simulink library "passive_control"  (Simulink 7.1)
values from neighbouring files (symbols this model uses):
  sysdsp = feedback(sysdp,Kc)    [calc_sysdsp.m]
  Ts = 1    [calc_sysdsp.m]
undefined symbols (not defined in the file or in its folder): A, B, b, C, D, gravload, Kv, Kx, M, ms, nc, np, q0, tau_passify
libraries: instrumentlib x8, passive_control x4, simulink x4, roblocks x2, dspsigops x2
(part 1 of 2)
settings Model: Creator=Administrator  LastModifiedBy=Tilt_Press

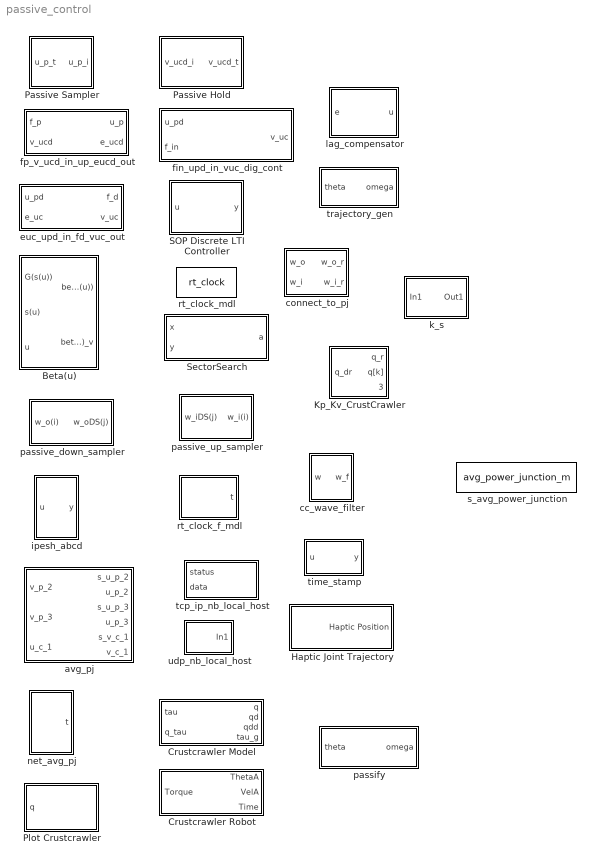
== system passive_control ==
  Beta(u) : Subsystem  mask{n=1}
      mask prompts: n "Enter Length of u"
  Crustcrawler Model : Subsystem  mask{q0=[0,-pi/2,pi/2,0]}
      mask prompts: q0 "Initial State [q0]"
      mask init:
      | srobot = crust_crawler_robot();
  Crustcrawler Robot : Subsystem  mask{Ts=0}
      mask prompts: Ts "Enter Ts"
  Haptic Joint Trajectory : Subsystem  SystemSampleTime=.04
  Kp_Kv_CrustCrawler : Subsystem  mask{q0=q0, Ts=Ts, Kv=Kv, Kx=Kx, Kg_on=off, b=b}
      mask prompts: q0 "Initial State (radians) [q0]"; Ts "Sample Rate (s) [Ts]"; Kv "Velocity Loop Gain [Kv]"; Kx "Position Loop Gain [Kx]"; Kg_on "Gravity Comp On [Kg] {0,1}"; b "wave impedance [b]"
      mask init:
      | if Kg_on
      |     Kg=1;
      | else
      |     Kg=0;
      | end
  Passive Hold : Subsystem  mask{Ts=.05}
      mask prompts: Ts "Hold Time (seconds):"
  Passive Sampler : Subsystem  mask{Ts=.05}
      mask prompts: Ts "Sample Time (seconds):"
  Plot Crustcrawler : Subsystem
      mask init:
      | srobot = crust_crawler_robot();
  SOP Discrete LTI Controller : Subsystem  mask{Kp=1, Kd=1, Kc=1.0e-6, x0=0, Ts=.05}
      mask prompts: Kp "Enter Kp (Kp > 0), (Kp in R^(mxm)):"; Kd "Enter Kd (Kd > 0), (Kd in R^(mxm)):"; Kc "Enter SOP feedback gain (Kc)"; x0 "Initial Conditions:"; Ts "Enter Sample Time (seconds):"
      mask help:
      | This will implement a (strictly) output passive digital controller
      | (if Kc > 0) based on its continuous passive PD controller counterpart.
      | The user just needs to insure that Kp > 0 and Kd > 0 (are positive
      | definite matrices).  For simplicity Kc can be a scalar.
      mask init:
      | [x0,sysdsp]=calc_sysdsp(Kp,Kd,Kc,x0,Ts);
  SectorSearch : Subsystem
  avg_pj : Subsystem  Orientation=left  mask{np=2, nc=1, ms=3, Ts=.05}
      mask prompts: np "Enter Number of Plants [np]"; nc "Enter Number of Controllers [nc]"; ms "Enter Vector Length [ms]"; Ts "Enter Sample Time (s) [Ts]"
  cc_wave_filter : Subsystem  mask{wn=1, Ts=.04}
      mask prompts: wn "Enter wn [wn] (rad/sec)"; Ts "Enter Sample rate [Ts] (sec)"
  connect_to_pj : Subsystem  mask{connect=on}
  euc_upd_in_fd_vuc_out : Subsystem  mask{b=1}
      mask prompts: b "Enter b:"
  fin_upd_in_vuc_dig_cont : Subsystem  mask{Kp=1, Kd=1, Kc=1.0e-6, b=1, x0=0, Ts=.05}
      mask prompts: Kp "Enter Kp (Kp > 0), (Kp in R^(mxm)):"; Kd "Enter Kd (Kd > 0), (Kd in R^(mxm)):"; Kc "Enter SOP feedback gain (Kc):"; b "Enter b:"; x0 "Initial Conditions:"; Ts "Enter Sample Time (seconds):"
      mask init:
      | [x0,sysdsp]=calc_sysdsp(Kp,Kd,Kc,x0,Ts);
      | sysdsp_ib=feedback(sysdsp,(1/b)*eye(size(sysdsp.d)));
  fp_v_ucd_in_up_eucd_out : Subsystem  mask{b=1}
      mask prompts: b "Enter b:"
  ipesh_abcd : Subsystem  mask{num=[1 0], den=[.02/pi 1], Ts=.02}
      mask prompts: num "Enter num of H(s) [num]"; den "Enter den of H(s) [den]"; Ts "Enter sample time (s) [Ts]"
      mask init:
      | Hs=tf(num,den);
      | Hz=ipesh_transform(Hs,Ts);
      | [A,B,C,D]=tf2ss(Hz.num{1},Hz.den{1});
      | [m,n]=size(A);
      | x0=zeros(1,n);
  k_s : Subsystem  mask{M=2, n_p=2}
      mask prompts: M "Enter Upsample / Downsample [M]"; n_p "Enter number of plants"
      mask init:
      | m=1;
      | n=n_p+m;
      | k_s=sqrt(M)*sqrt((n-m))/sqrt(m);
  lag_compensator : Subsystem  mask{K=.5, omega=pi/2, Ts=2*.04}
      mask prompts: omega "omega (rad/sec) [omega]"; Ts "sample rate (s) [Ts]"
  net_avg_pj : Subsystem  mask{udp_start_port=9000, Ts=.05, max_pc=100, ID=1}
      mask prompts: udp_start_port "Enter UDP Start Port [udp_start_port]"; Ts "Enter PJ Sample Time [Ts]"; max_pc "Enter max_pc [max_pc]"; ID "Enter time ID [ID]"
      mask CallbackString:
      | udp_start_port=eval(get_param(gcb,'udp_start_port'));
      | max_pc=eval(get_param(gcb,'max_pc'));
      | Ts=eval(get_param(gcb,'Ts'));
      | for i = 2:3
      |     obj=[gcb,'/Plant_',num2str(i),'_u'];
      |     set_param(obj,'port',num2str(udp_start_port+max_pc+i-1));
      |     set_param(obj,'Ts',num2str(Ts));
      |     obj=[gcb,'/Plant_',num2str(i),'_v'];
      |     set_param(obj,'port',num2str(udp_start_port+2*max_pc+i-1));
      | end
      | set_param([gcb,'/Controller_1_v'],'port',num2str(udp_start_port+max_pc));
      | set_param([gcb,'/Controller_1_v'],'Ts',num2str(Ts));
      | set_param([gcb,'/Controller_1_u'],'port',num2str(udp_start_port+2*max_pc));
      | |||
  passify : Subsystem  mask{tau=tau_passify, Ts=Ts}
      mask prompts: tau "tau (seconds) [tau]"; Ts "Sample rate (seconds) Ts"
  passive_down_sampler : Subsystem  mask{M=M}
      mask prompts: M "Enter Downsample Integer M:"
  passive_up_sampler : Subsystem  mask{M=2, N=2}
      mask prompts: M "Enter Upsampler Integer M:"; N "Dimension of Input Vector N:"
  rt_clock_f_mdl : Subsystem  mask{Ts=.05, ID=1}
      mask prompts: Ts "Enter Step Size (seconds)"; ID "Enter Timer ID {1,2,...}"
  rt_clock_mdl : S-Function  FunctionName=rt_clock  Parameters=1,.05  EnableBusSupport=off
  s_avg_power_junction : S-Function  FunctionName=avg_power_junction_m  Parameters=ms,np,nc,Ts  EnableBusSupport=off
  tcp_ip_nb_local_host : Subsystem  Orientation=left  mask{port=10000, ms=3, Ts=.05}
      mask prompts: port "Port: [port]"; ms "Vector length: [ms]"; Ts "Block sample time: [Ts]"
      mask CallbackString:
      | port=eval(get_param(gcb,'port'));
      | set_param([gcb,'/tcp_ip_r'],'Port',num2str(port));
      | |ms=eval(get_param(gcb,'ms'));
      | set_param([gcb,'/tcp_ip_r'],'DataSize',['[',num2str(ms),']']);|Ts=eval(get_param(gcb,'Ts'));
      | set_param([gcb,'/tcp_ip_r'],'SampleTime',num2str(Ts));
  time_stamp : Subsystem
      mask Description:
      | Adds return from clock to vector, to plot results which
      | were stored to file plant.mat for example do the following:
      | fh=load('plant');
      | t=fh.ans(1,:);
      | c_v=fh.ans(2:7,:);
      | theta=fh.ans(8:11,:);
      | t_ts=0*t;
      | i=1;
      | c_0=c_v(:,1);
      | for c = c_v
      |     t_ts(i) = etime(c',c_0');
      |     i = i + 1;
      | end
      | plot(t_ts,t-t_ts,t_ts,theta);grid;
  trajectory_gen : Subsystem  mask{zeta=.9, wn=2*pi/10, Ts=2*.04}
      mask prompts: zeta "zeta [zeta]"; wn "wn [wn] (rad/sec)"; Ts "sample rate (s) [Ts]"
  udp_nb_local_host : Subsystem  Orientation=left  mask{port=9001}
      mask prompts: port "Port: [port]"
      mask CallbackString:
      | port=eval(get_param(gcb,'port'));
      | set_param([gcb,'/udp_s'],'Port',num2str(port));

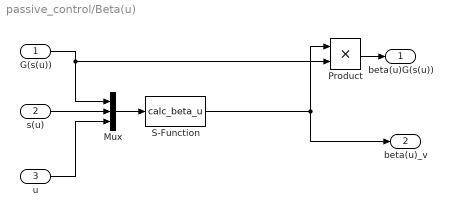
== system passive_control/Beta(u) ==
  G(s(u)) : Inport  OutDataType=sfix(16)  OutScaling=2^0
  s(u) : Inport  Port=2  OutDataType=sfix(16)  OutScaling=2^0
  u : Inport  Port=3  OutDataType=sfix(16)  OutScaling=2^0
  Mux : Mux  Inputs=3
  Product : Product  OutDataType=sfix(16)  OutScaling=2^0  RndMeth=Zero
  S-Function : S-Function  FunctionName=calc_beta_u  Parameters=n  EnableBusSupport=off
  beta(u)G(s(u)) : Outport  OutDataType=sfix(16)  OutScaling=2^0
  beta(u)_v : Outport  Port=2  OutDataType=sfix(16)  OutScaling=2^0
  wires:
  Product/1 -> beta(u)G(s(u))/1
  Mux/1 -> S-Function/1
  u/1 -> Mux/3
  s(u)/1 -> Mux/2
  G(s(u))/1 -> Product/2, Mux/1
  S-Function/1 -> Product/1, beta(u)_v/1

== system passive_control/Crustcrawler Model ==
  tau : Inport  OutDataType=sfix(16)  OutScaling=2^0
  q_tau : Inport  Port=2  OutDataType=sfix(16)  OutScaling=2^0
  Robot : roblocks/Robot  SystemSampleTime=-1  robot=srobot  q0=q0
      link override Integrator1: InitialCondition=q0
  gravity_compensation : MATLABFcn  MATLABFcn=gravload(srobot, u(1:4)')  OutputDimensions=4
  q : Outport  OutDataType=sfix(16)  OutScaling=2^0
  qd : Outport  Port=2  OutDataType=sfix(16)  OutScaling=2^0
  qdd : Outport  Port=3  OutDataType=sfix(16)  OutScaling=2^0
  tau_g : Outport  Port=4  OutDataType=sfix(16)  OutScaling=2^0
  wires:
  q_tau/1 -> gravity_compensation/1
  gravity_compensation/1 -> tau_g/1
  tau/1 -> Robot/1
  Robot/1 -> q/1
  Robot/2 -> qd/1
  Robot/3 -> qdd/1

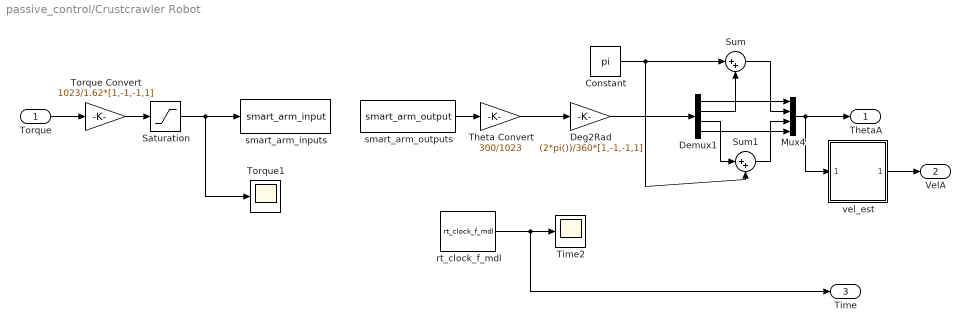
== system passive_control/Crustcrawler Robot ==
  Torque : Inport
  Constant : Constant  Value=pi  OutDataType=sfix(16)  OutScaling=2^0  SampleTime=Ts
  Deg2Rad : Gain  Gain=(2*pi())/360*[1,-1,-1,1]  ParameterDataType=sfix(16)  ParameterScaling=2^0  OutDataType=sfix(16)  OutScaling=2^0
  Demux1 : Demux
  Mux4 : Mux
  Saturation : Saturate  UpperLimit=1023  LowerLimit=-1023  OutDataType=sfix(16)  OutScaling=2^0
  Sum : Sum  Inputs=|++  OutDataType=sfix(16)  OutScaling=2^0
  Sum1 : Sum  Inputs=|++  OutDataType=sfix(16)  OutScaling=2^0
  Theta Convert : Gain  Gain=300/1023  ParameterDataType=sfix(16)  ParameterScaling=2^0  OutDataType=sfix(16)  OutScaling=2^0
  Time2 : Scope
      settings: TimeRange=100  YMin=-0.0275  YMax=0.02
  Torque Convert : Gain  Gain=1023/1.62*[1,-1,-1,1]  ParameterDataType=sfix(16)  ParameterScaling=2^0  OutDataType=sfix(16)  OutScaling=2^0
  Torque1 : Scope
      settings: TimeRange=100  YMin=-175  YMax=375
  rt_clock_f_mdl : passive_control/rt_clock_f_mdl  SystemSampleTime=-1  Ts=Ts  ID=1
  smart_arm_inputs : S-Function  Priority=1  FunctionName=smart_arm_input  Parameters=1, Ts  EnableBusSupport=off
  smart_arm_outputs : S-Function  Priority=2  FunctionName=smart_arm_output  Parameters=1, Ts  EnableBusSupport=off
  vel_est : Subsystem
  ThetaA : Outport
  VelA : Outport  Port=2
  Time : Outport  Port=3
  wires:
  vel_est/1(omega) -> VelA/1
  rt_clock_f_mdl/1 -> Time/1, Time2/1
  Torque/1 -> Torque Convert/1
  Theta Convert/1 -> Deg2Rad/1
  Torque Convert/1 -> Saturation/1
  Mux4/1 -> vel_est/1(theta), ThetaA/1
  Demux1/1 -> Mux4/1
  Demux1/4 -> Mux4/4
  Deg2Rad/1 -> Demux1/1
  Sum/1 -> Mux4/2
  Constant/1 -> Sum/1, Sum1/2
  Demux1/2 -> Sum/2
  Demux1/3 -> Sum1/1
  Sum1/1 -> Mux4/3
  smart_arm_outputs/1 -> Theta Convert/1
  Saturation/1 -> Torque1/1, smart_arm_inputs/1

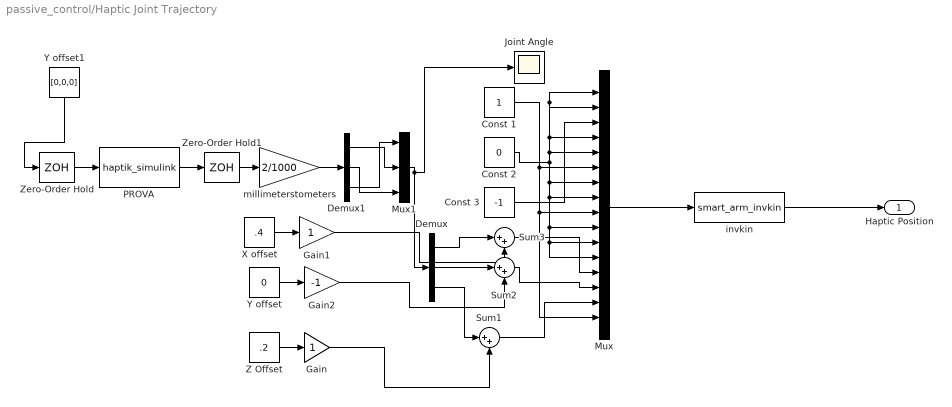
== system passive_control/Haptic Joint Trajectory ==
  Const 1 : Constant  OutDataType=sfix(16)  OutScaling=2^0
  Const 2 : Constant  Value=0  OutDataType=sfix(16)  OutScaling=2^0
  Const 3 : Constant  Value=-1  OutDataType=sfix(16)  OutScaling=2^0
  Demux : Demux  Outputs=3
  Demux1 : Demux  Outputs=3
  Gain : Gain  ParameterDataType=sfix(16)  ParameterScaling=2^0  OutDataType=sfix(16)  OutScaling=2^0
  Gain1 : Gain  ParameterDataType=sfix(16)  ParameterScaling=2^0  OutDataType=sfix(16)  OutScaling=2^0
  Gain2 : Gain  Gain=-1  ParameterDataType=sfix(16)  ParameterScaling=2^0  OutDataType=sfix(16)  OutScaling=2^0
  Joint Angle : Scope
      settings: TimeRange=100  YMin=-0.06  YMax=0.015
  Mux : Mux  Inputs=16
  Mux1 : Mux  Inputs=3
  PROVA : S-Function  FunctionName=haptik_simulink  EnableBusSupport=off
  Sum1 : Sum  Inputs=|++  OutDataType=sfix(16)  OutScaling=2^0
  Sum2 : Sum  Inputs=|++  OutDataType=sfix(16)  OutScaling=2^0
  Sum3 : Sum  Inputs=|++  OutDataType=sfix(16)  OutScaling=2^0
  X offset : Constant  Value=.4  OutDataType=sfix(16)  OutScaling=2^0
  Y offset : Constant  Value=0  OutDataType=sfix(16)  OutScaling=2^0
  Y offset1 : Constant  Orientation=down  Value=[0,0,0]  OutDataType=sfix(16)  OutScaling=2^0
  Z Offset : Constant  Value=.2  OutDataType=sfix(16)  OutScaling=2^0
  Zero-Order Hold : ZeroOrderHold  SampleTime=.04
  Zero-Order Hold1 : ZeroOrderHold  SampleTime=.04
  invkin : S-Function  FunctionName=smart_arm_invkin  Parameters=1  EnableBusSupport=off
  millimeterstometers : Gain  Gain=2/1000  ParameterDataType=sfix(16)  ParameterScaling=2^0  OutDataType=sfix(16)  OutScaling=2^0
  Haptic Position : Outport  OutDataType=sfix(16)  OutScaling=2^0
  wires:
  Gain1/1 -> Sum3/2
  Sum3/1 -> Mux/13
  Demux/1 -> Sum3/1
  X offset/1 -> Gain1/1
  Gain2/1 -> Sum2/2
  Sum2/1 -> Mux/14
  Demux/2 -> Sum2/1
  Mux1/1 -> Joint Angle/1, Demux/1
  millimeterstometers/1 -> Demux1/1
  Mux/1 -> invkin/1
  Const 2/1 -> Mux/4, Mux/1, Mux/2, Mux/5, Mux/8, Mux/10, Mux/12, Mux/11, Mux/7
  Const 1/1 -> Mux/6, Mux/16, Mux/9
  Sum1/1 -> Mux/15
  Gain/1 -> Sum1/2
  Demux/3 -> Sum1/1
  Z Offset/1 -> Gain/1
  Y offset/1 -> Gain2/1
  PROVA/1 -> Zero-Order Hold1/1
  Const 3/1 -> Mux/3
  Demux1/2 -> Mux1/3
  Demux1/1 -> Mux1/2
  Demux1/3 -> Mux1/1
  Zero-Order Hold/1 -> PROVA/1
  Zero-Order Hold1/1 -> millimeterstometers/1
  Y offset1/1 -> Zero-Order Hold/1
  invkin/1 -> Haptic Position/1

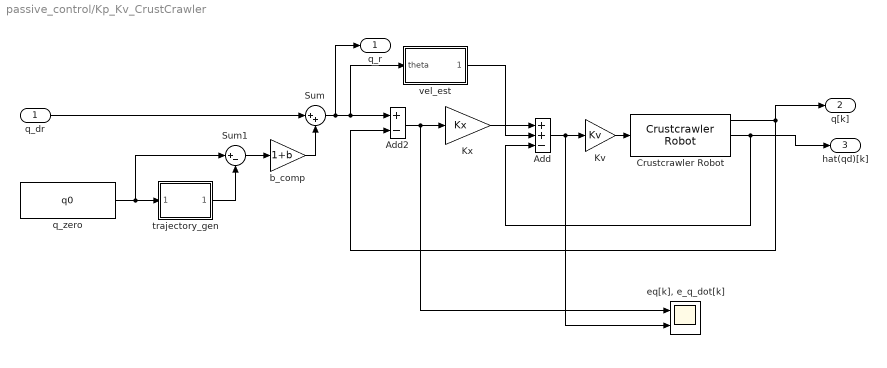
== system passive_control/Kp_Kv_CrustCrawler ==
  q_dr : Inport
  Add : Sum  Inputs=++-  OutDataType=sfix(16)  OutScaling=2^-10
  Add2 : Sum  Inputs=+-  OutDataType=sfix(16)  OutScaling=2^-10
  Crustcrawler Robot : passive_control/Crustcrawler Robot  SystemSampleTime=-1  Ts=Ts
  Kv : Gain  Gain=Kv  ParameterDataType=sfix(16)  ParameterScaling=2^0  OutDataType=sfix(16)  OutScaling=2^0
  Kx : Gain  Gain=Kx  ParameterDataType=sfix(16)  ParameterScaling=2^0  OutDataType=sfix(16)  OutScaling=2^0
  Sum : Sum  Inputs=|++  OutDataType=sfix(16)  OutScaling=2^0
  Sum1 : Sum  Inputs=|+-  OutDataType=sfix(16)  OutScaling=2^0
  b_comp : Gain  Gain=1+b  ParameterDataType=sfix(16)  ParameterScaling=2^0  OutDataType=sfix(16)  OutScaling=2^0
  "eq[k], e_q_dot[k]" : Scope  NumInputPorts=2
      settings: TimeRange=5  YMin=-0.01~-0.2  YMax=0.035~1  SaveName=ScopeData5
  q_zero : Constant  Value=q0  OutDataType=sfix(16)  OutScaling=2^0  SampleTime=0.04
  trajectory_gen : Subsystem  mask{zeta=.9, wn=2*pi/10, Ts=Ts}
      mask prompts: zeta "zeta [zeta]"; wn "wn [wn] (rad/sec)"; Ts "sample rate (s) [Ts]"
  vel_est : Subsystem  Priority=-1  mask{Ts=Ts, q0=q0*(1+b)}
      mask prompts: Ts "Enter Sample Rate [Ts] (seconds)"; q0 "Enter Initial State [q0] (radians)"
  q_r : Outport
  q[k] : Outport  Port=2
  hat(qd)[k] : Outport  Port=3
  wires:
  vel_est/1(omega) -> Add/2
  q_dr/1 -> Sum/1
  Crustcrawler Robot/2 -> hat(qd)[k]/1, Add/3
  Crustcrawler Robot/1 -> q[k]/1, Add2/2
  Sum/1 -> q_r/1, vel_est/1(theta), Add2/1
  Add/1 -> "eq[k], e_q_dot[k]"/2, Kv/1
  Kv/1 -> Crustcrawler Robot/1
  Kx/1 -> Add/1
  Add2/1 -> "eq[k], e_q_dot[k]"/1, Kx/1
  trajectory_gen/1(omega) -> Sum1/2
  q_zero/1 -> Sum1/1, trajectory_gen/1(theta)
  Sum1/1 -> b_comp/1
  b_comp/1 -> Sum/2

== system passive_control/Passive Hold ==
  v_ucd_i : Inport  OutDataType=sfix(16)  OutScaling=2^0
  Gain : Gain  Gain=1/sqrt(Ts)  ParameterDataType=sfix(16)  ParameterScaling=2^0  OutDataType=sfix(16)  OutScaling=2^0
  Zero-Order Hold : ZeroOrderHold  SampleTime=Ts
  v_ucd_t : Outport  OutDataType=sfix(16)  OutScaling=2^0
  wires:
  Zero-Order Hold/1 -> Gain/1
  Gain/1 -> v_ucd_t/1
  v_ucd_i/1 -> Zero-Order Hold/1

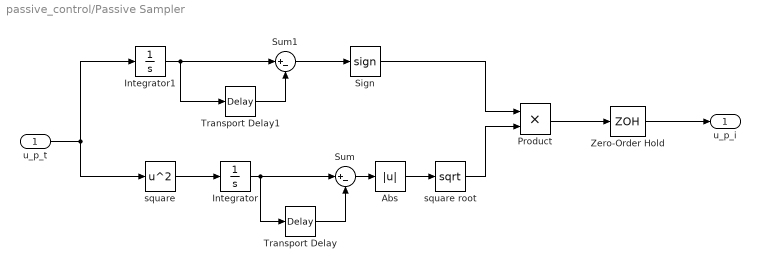
== system passive_control/Passive Sampler ==
  u_p_t : Inport  OutDataType=sfix(16)  OutScaling=2^0
  Abs : Abs  OutDataType=sfix(16)  OutScaling=2^0
  Integrator : Integrator
  Integrator1 : Integrator
  Product : Product  OutDataType=sfix(16)  OutScaling=2^0  RndMeth=Zero
  Sign : Signum
  Sum : Sum  Inputs=|+-  OutDataType=sfix(16)  OutScaling=2^0
  Sum1 : Sum  Inputs=|+-  OutDataType=sfix(16)  OutScaling=2^0
  Transport Delay : TransportDelay  DelayTime=Ts
  Transport Delay1 : TransportDelay  DelayTime=Ts
  Zero-Order Hold : ZeroOrderHold  SampleTime=Ts
  square : Math  Operator=square  OutDataType=sfix(16)  OutScaling=2^0  SaturateOnIntegerOverflow=on
  square root : Math  Operator=sqrt  OutDataType=sfix(16)  OutScaling=2^0  SaturateOnIntegerOverflow=on
  u_p_i : Outport  OutDataType=sfix(16)  OutScaling=2^0
  wires:
  Transport Delay/1 -> Sum/2
  Transport Delay1/1 -> Sum1/2
  Zero-Order Hold/1 -> u_p_i/1
  Sum1/1 -> Sign/1
  Integrator1/1 -> Sum1/1, Transport Delay1/1
  Sum/1 -> Abs/1
  Integrator/1 -> Transport Delay/1, Sum/1
  Sign/1 -> Product/1
  square root/1 -> Product/2
  square/1 -> Integrator/1
  u_p_t/1 -> square/1, Integrator1/1
  Abs/1 -> square root/1
  Product/1 -> Zero-Order Hold/1

== system passive_control/Plot Crustcrawler ==
  q : Inport  OutDataType=sfix(16)  OutScaling=2^0
  plot : roblocks/plot  SystemSampleTime=-1  robot=srobot
  wires:
  q/1 -> plot/1

== system passive_control/SOP Discrete LTI Controller ==
  u : Inport  OutDataType=sfix(16)  OutScaling=2^0
  Discrete State-Space : DiscreteStateSpace  A=sysdsp.a  B=sysdsp.b  C=sysdsp.c  D=sysdsp.d  X0=x0  SampleTime=-1
  y : Outport  OutDataType=sfix(16)  OutScaling=2^0
  wires:
  u/1 -> Discrete State-Space/1
  Discrete State-Space/1 -> y/1

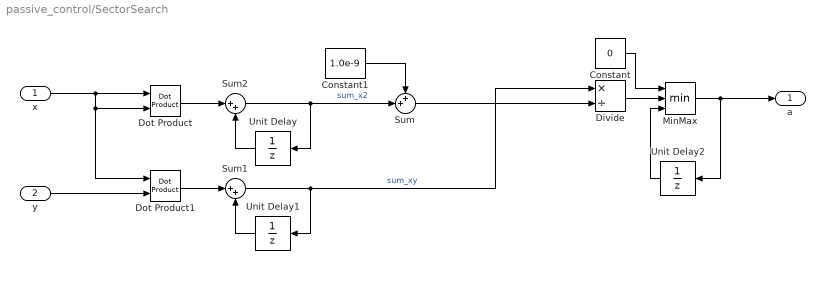
== system passive_control/SectorSearch ==
  x : Inport  OutDataType=sfix(16)  OutScaling=2^0
  y : Inport  Port=2  OutDataType=sfix(16)  OutScaling=2^0
  Constant : Constant  Value=0  OutDataType=sfix(16)  OutScaling=2^0
  Constant1 : Constant  Value=1.0e-9  OutDataType=sfix(16)  OutScaling=2^0
  Divide : Product  Inputs=*/  OutDataType=sfix(16)  OutScaling=2^-10
  Dot Product : simulink/Math Operations/Dot Product  InputSameDT=on  OutDataType=sfix(16)  OutScaling=2^-10  DoSatur=off
  Dot Product1 : simulink/Math Operations/Dot Product  InputSameDT=on  OutDataType=sfix(16)  OutScaling=2^-10  DoSatur=off
  MinMax : MinMax  Inputs=3  OutDataType=sfix(16)  OutScaling=2^0
  Sum : Sum  Inputs=++|  OutDataType=sfix(16)  OutScaling=2^0
  Sum1 : Sum  Inputs=|++  OutDataType=sfix(16)  OutScaling=2^0
  Sum2 : Sum  Inputs=|++  OutDataType=sfix(16)  OutScaling=2^0
  Unit Delay : UnitDelay  Orientation=left  SampleTime=-1
  Unit Delay1 : UnitDelay  Orientation=left  SampleTime=-1
  Unit Delay2 : UnitDelay  Orientation=left  SampleTime=-1
  a : Outport  OutDataType=sfix(16)  OutScaling=2^0
  wires:
  Sum2/1 -> Unit Delay/1, Sum/2  "sum_x2"
  Unit Delay/1 -> Sum2/2
  Dot Product/1 -> Sum2/1
  Sum1/1 -> Unit Delay1/1, Divide/1  "sum_xy"
  Unit Delay1/1 -> Sum1/2
  Dot Product1/1 -> Sum1/1
  x/1 -> Dot Product/1, Dot Product/2, Dot Product1/1
  y/1 -> Dot Product1/2
  MinMax/1 -> Unit Delay2/1, a/1
  Constant/1 -> MinMax/1
  Divide/1 -> MinMax/2
  Unit Delay2/1 -> MinMax/3
  Sum/1 -> Divide/2
  Constant1/1 -> Sum/1

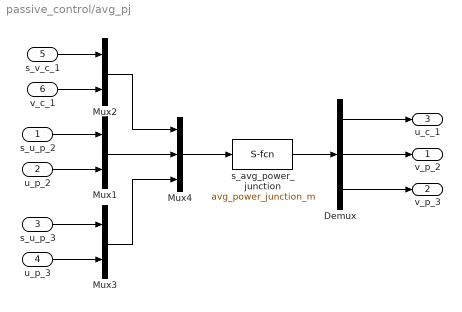
== system passive_control/avg_pj ==
  s_u_p_2 : Inport
  u_p_2 : Inport  Port=2
  s_u_p_3 : Inport  Port=3
  u_p_3 : Inport  Port=4
  s_v_c_1 : Inport  Port=5
  v_c_1 : Inport  Port=6
  Demux : Demux  Outputs=3
  Mux1 : Mux  Inputs=2
  Mux2 : Mux  Inputs=2
  Mux3 : Mux  Inputs=2
  Mux4 : Mux  Inputs=3
  s_avg_power_junction : S-Function  FunctionName=avg_power_junction_m  Parameters=ms,np,nc,Ts  EnableBusSupport=off
  v_p_2 : Outport
  v_p_3 : Outport  Port=2
  u_c_1 : Outport  Port=3
  wires:
  s_avg_power_junction/1 -> Demux/1
  Mux4/1 -> s_avg_power_junction/1
  Demux/3 -> v_p_3/1
  Demux/2 -> v_p_2/1
  Demux/1 -> u_c_1/1
  Mux3/1 -> Mux4/3
  Mux1/1 -> Mux4/2
  Mux2/1 -> Mux4/1
  u_p_3/1 -> Mux3/2
  s_u_p_3/1 -> Mux3/1
  u_p_2/1 -> Mux1/2
  s_u_p_2/1 -> Mux1/1
  v_c_1/1 -> Mux2/2
  s_v_c_1/1 -> Mux2/1

== system passive_control/cc_wave_filter ==
  w : Inport
  Demux : Demux
  Mux : Mux
  ipesh_abcd : Subsystem  AncestorBlock=passive_control/ipesh_abcd  mask{num=[wn^2], den=[1,2*wn,wn^2], Ts=Ts}
      mask prompts: num "Enter num of H(s) [num]"; den "Enter den of H(s) [den]"; Ts "Enter sample time (s) [Ts]"
      mask init:
      | Hs=tf(num,den);
      | Hz=ipesh_transform(Hs,Ts);
      | [A,B,C,D]=tf2ss(Hz.num{1},Hz.den{1});
      | [m,n]=size(A);
      | x0=zeros(1,n);
  ipesh_abcd1 : Subsystem  AncestorBlock=passive_control/ipesh_abcd  mask{num=[wn^2], den=[1,2*wn,wn^2], Ts=Ts}
      mask prompts: num "Enter num of H(s) [num]"; den "Enter den of H(s) [den]"; Ts "Enter sample time (s) [Ts]"
      mask init:
      | Hs=tf(num,den);
      | Hz=ipesh_transform(Hs,Ts);
      | [A,B,C,D]=tf2ss(Hz.num{1},Hz.den{1});
      | [m,n]=size(A);
      | x0=zeros(1,n);
  ipesh_abcd2 : Subsystem  AncestorBlock=passive_control/ipesh_abcd  mask{num=[wn^2], den=[1,2*wn,wn^2], Ts=Ts}
      mask prompts: num "Enter num of H(s) [num]"; den "Enter den of H(s) [den]"; Ts "Enter sample time (s) [Ts]"
      mask init:
      | Hs=tf(num,den);
      | Hz=ipesh_transform(Hs,Ts);
      | [A,B,C,D]=tf2ss(Hz.num{1},Hz.den{1});
      | [m,n]=size(A);
      | x0=zeros(1,n);
  ipesh_abcd3 : Subsystem  AncestorBlock=passive_control/ipesh_abcd  mask{num=[wn^2], den=[1,2*wn,wn^2], Ts=Ts}
      mask prompts: num "Enter num of H(s) [num]"; den "Enter den of H(s) [den]"; Ts "Enter sample time (s) [Ts]"
      mask init:
      | Hs=tf(num,den);
      | Hz=ipesh_transform(Hs,Ts);
      | [A,B,C,D]=tf2ss(Hz.num{1},Hz.den{1});
      | [m,n]=size(A);
      | x0=zeros(1,n);
  w_f : Outport
  wires:
  ipesh_abcd3/1(y) -> Mux/4
  Demux/4 -> ipesh_abcd3/1(u)
  ipesh_abcd2/1(y) -> Mux/3
  Demux/3 -> ipesh_abcd2/1(u)
  ipesh_abcd1/1(y) -> Mux/2
  Demux/2 -> ipesh_abcd1/1(u)
  ipesh_abcd/1(y) -> Mux/1
  Demux/1 -> ipesh_abcd/1(u)
  w/1 -> Demux/1
  Mux/1 -> w_f/1

== system passive_control/connect_to_pj ==
  w_o : Inport
  w_i : Inport  Port=2
  connect_to_pj : Stateflow chart
  w_o_r : Outport
  w_i_r : Outport  Port=2
  wires:
  w_o/1 -> connect_to_pj/1(w_o)
  w_i/1 -> connect_to_pj/2(w_i)
  connect_to_pj/1(w_o_r) -> w_o_r/1
  connect_to_pj/2(w_i_r) -> w_i_r/1

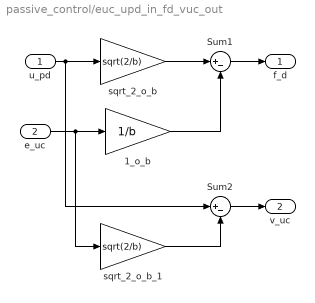
== system passive_control/euc_upd_in_fd_vuc_out ==
  u_pd : Inport  OutDataType=sfix(16)  OutScaling=2^0
  e_uc : Inport  Port=2  OutDataType=sfix(16)  OutScaling=2^0
  1_o_b : Gain  Gain=1/b  ParameterDataType=sfix(16)  ParameterScaling=2^0  OutDataType=sfix(16)  OutScaling=2^0
  Sum1 : Sum  Inputs=|+-  OutDataType=sfix(16)  OutScaling=2^0
  Sum2 : Sum  Inputs=|+-  OutDataType=sfix(16)  OutScaling=2^0
  sqrt_2_o_b : Gain  Gain=sqrt(2/b)  ParameterDataType=sfix(16)  ParameterScaling=2^0  OutDataType=sfix(16)  OutScaling=2^0
  sqrt_2_o_b_1 : Gain  Gain=sqrt(2/b)  ParameterDataType=sfix(16)  ParameterScaling=2^0  OutDataType=sfix(16)  OutScaling=2^0
  f_d : Outport  OutDataType=sfix(16)  OutScaling=2^0
  v_uc : Outport  Port=2  OutDataType=sfix(16)  OutScaling=2^0
  wires:
  u_pd/1 -> sqrt_2_o_b/1, Sum2/1
  Sum1/1 -> f_d/1
  sqrt_2_o_b/1 -> Sum1/1
  e_uc/1 -> 1_o_b/1, sqrt_2_o_b_1/1
  1_o_b/1 -> Sum1/2
  sqrt_2_o_b_1/1 -> Sum2/2
  Sum2/1 -> v_uc/1

== system passive_control/fin_upd_in_vuc_dig_cont ==
  u_pd : Inport  OutDataType=sfix(16)  OutScaling=2^0
  f_in : Inport  Port=2  OutDataType=sfix(16)  OutScaling=2^0
  Discrete State-Space : DiscreteStateSpace  A=sysdsp_ib.a  B=sysdsp_ib.b  C=sysdsp_ib.c  D=sysdsp_ib.d  SampleTime=-1
  Gain : Gain  Orientation=up  Gain=sqrt(2/b)  ParameterDataType=sfix(16)  ParameterScaling=2^0  OutDataType=sfix(16)  OutScaling=2^0
  Gain1 : Gain  Orientation=down  Gain=sqrt(2/b)  ParameterDataType=sfix(16)  ParameterScaling=2^0  OutDataType=sfix(16)  OutScaling=2^0
  Sum1 : Sum  Inputs=|++  OutDataType=sfix(16)  OutScaling=2^0
  Sum2 : Sum  Orientation=down  Inputs=+-|  OutDataType=sfix(16)  OutScaling=2^0
  v_uc : Outport  OutDataType=sfix(16)  OutScaling=2^0
  wires:
  f_in/1 -> Sum1/1
  Sum1/1 -> Discrete State-Space/1
  u_pd/1 -> Gain/1, Sum2/1
  Gain/1 -> Sum1/2
  Discrete State-Space/1 -> Gain1/1
  Gain1/1 -> Sum2/2
  Sum2/1 -> v_uc/1

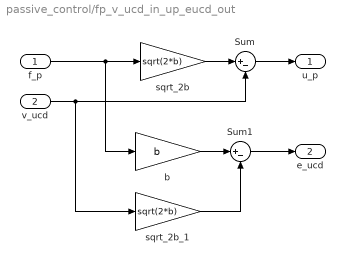
== system passive_control/fp_v_ucd_in_up_eucd_out ==
  f_p : Inport  OutDataType=sfix(16)  OutScaling=2^0
  v_ucd : Inport  Port=2  OutDataType=sfix(16)  OutScaling=2^0
  Sum : Sum  Inputs=|+-  OutDataType=sfix(16)  OutScaling=2^0
  Sum1 : Sum  Inputs=|+-  OutDataType=sfix(16)  OutScaling=2^0
  b : Gain  Gain=b  ParameterDataType=sfix(16)  ParameterScaling=2^0  OutDataType=sfix(16)  OutScaling=2^0
  sqrt_2b : Gain  Gain=sqrt(2*b)  ParameterDataType=sfix(16)  ParameterScaling=2^0  OutDataType=sfix(16)  OutScaling=2^0
  sqrt_2b_1 : Gain  Gain=sqrt(2*b)  ParameterDataType=sfix(16)  ParameterScaling=2^0  OutDataType=sfix(16)  OutScaling=2^0
  u_p : Outport  OutDataType=sfix(16)  OutScaling=2^0
  e_ucd : Outport  Port=2  OutDataType=sfix(16)  OutScaling=2^0
  wires:
  f_p/1 -> sqrt_2b/1, b/1
  Sum/1 -> u_p/1
  v_ucd/1 -> Sum/2, sqrt_2b_1/1
  sqrt_2b/1 -> Sum/1
  b/1 -> Sum1/1
  Sum1/1 -> e_ucd/1
  sqrt_2b_1/1 -> Sum1/2

== system passive_control/ipesh_abcd ==
  u : Inport
  Embedded MATLAB Function : Stateflow chart
  Unit Delay : UnitDelay  Orientation=left  X0=x0  SampleTime=-1
  y : Outport
  wires:
  Embedded MATLAB Function/1(y) -> y/1
  u/1 -> Embedded MATLAB Function/1(u)
  Unit Delay/1 -> Embedded MATLAB Function/2(x_k)
  Embedded MATLAB Function/2(x_k_p_1) -> Unit Delay/1

== system passive_control/k_s ==
  In1 : Inport
  k_s : Gain  Gain=-k_s  ParameterDataType=sfix(16)  ParameterScaling=2^0  OutDataType=sfix(16)  OutScaling=2^0
  Out1 : Outport
  wires:
  In1/1 -> k_s/1
  k_s/1 -> Out1/1

== system passive_control/lag_compensator ==
  e : Inport
  Demux3 : Demux
  Mux7 : Mux
  lag_compen : Subsystem  AncestorBlock=passive_control/ipesh_abcd  mask{num=K*[1,omega], den=[1,0], Ts=Ts, xp0=[0,0]}
      mask prompts: num "Enter num of H(s) [num]"; den "Enter den of H(s) [den]"; Ts "Enter sample time (s) [Ts]"; xp0 "Initial Joint Angle [xp0]"
      mask init:
      | Hs=tf(num,den);
      | Hz=ipesh_transform(Hs,Ts);
      | [A,B,C,D]=tf2ss(Hz.num{1},Hz.den{1})
      | [m,n]=size(A);
      | x0=zeros(n,1);
  lag_compen1 : Subsystem  AncestorBlock=passive_control/ipesh_abcd  mask{num=K*[1,omega], den=[1,0], Ts=Ts, xp0=[0,0]}
      mask prompts: num "Enter num of H(s) [num]"; den "Enter den of H(s) [den]"; Ts "Enter sample time (s) [Ts]"; xp0 "Initial Joint Angle [xp0]"
      mask init:
      | Hs=tf(num,den);
      | Hz=ipesh_transform(Hs,Ts);
      | [A,B,C,D]=tf2ss(Hz.num{1},Hz.den{1})
      | [m,n]=size(A);
      | x0=zeros(n,1);
  lag_compen2 : Subsystem  AncestorBlock=passive_control/ipesh_abcd  mask{num=K*[1,omega], den=[1,0], Ts=Ts, xp0=[0,0]}
      mask prompts: num "Enter num of H(s) [num]"; den "Enter den of H(s) [den]"; Ts "Enter sample time (s) [Ts]"; xp0 "Initial Joint Angle [xp0]"
      mask init:
      | Hs=tf(num,den);
      | Hz=ipesh_transform(Hs,Ts);
      | [A,B,C,D]=tf2ss(Hz.num{1},Hz.den{1})
      | [m,n]=size(A);
      | x0=zeros(n,1);
  lag_compen3 : Subsystem  AncestorBlock=passive_control/ipesh_abcd  mask{num=K*[1,omega], den=[1,0], Ts=Ts, xp0=[0,0]}
      mask prompts: num "Enter num of H(s) [num]"; den "Enter den of H(s) [den]"; Ts "Enter sample time (s) [Ts]"; xp0 "Initial Joint Angle [xp0]"
      mask init:
      | Hs=tf(num,den);
      | Hz=ipesh_transform(Hs,Ts);
      | [A,B,C,D]=tf2ss(Hz.num{1},Hz.den{1})
      | [m,n]=size(A);
      | x0=zeros(n,1);
  u : Outport
  wires:
  lag_compen3/1(y) -> Mux7/4
  lag_compen2/1(y) -> Mux7/3
  lag_compen1/1(y) -> Mux7/2
  lag_compen/1(y) -> Mux7/1
  Mux7/1 -> u/1
  e/1 -> Demux3/1
  Demux3/4 -> lag_compen3/1(u)
  Demux3/3 -> lag_compen2/1(u)
  Demux3/2 -> lag_compen1/1(u)
  Demux3/1 -> lag_compen/1(u)

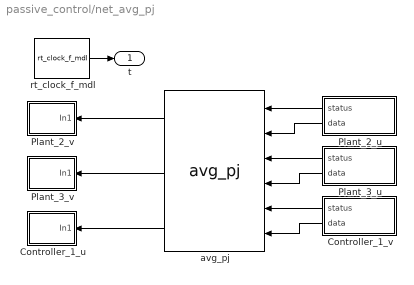
== system passive_control/net_avg_pj ==
  Controller_1_u : Subsystem  Orientation=left  AncestorBlock=passive_control/udp_nb_local_host  mask{port=9200}
      mask prompts: port "Port: [port]"
      mask CallbackString:
      | port=eval(get_param(gcb,'port'));
      | set_param([gcb,'/udp_s'],'Port',num2str(port));
  Controller_1_v : Subsystem  Orientation=left  AncestorBlock=passive_control/tcp_ip_nb_local_host  mask{port=9100, ms=3, Ts=0.05}
      mask prompts: port "Port: [port]"; ms "Vector length: [ms]"; Ts "Block sample time: [Ts]"
      mask CallbackString:
      | port=eval(get_param(gcb,'port'));
      | set_param([gcb,'/tcp_ip_r'],'Port',num2str(port));
      | |ms=eval(get_param(gcb,'ms'));
      | set_param([gcb,'/tcp_ip_r'],'DataSize',['[',num2str(ms),']']);|Ts=eval(get_param(gcb,'Ts'));
      | set_param([gcb,'/tcp_ip_r'],'SampleTime',num2str(Ts));
  Plant_2_u : Subsystem  Orientation=left  AncestorBlock=passive_control/tcp_ip_nb_local_host  mask{port=9101, ms=3, Ts=0.05}
      mask prompts: port "Port: [port]"; ms "Vector length: [ms]"; Ts "Block sample time: [Ts]"
      mask CallbackString:
      | port=eval(get_param(gcb,'port'));
      | set_param([gcb,'/tcp_ip_r'],'Port',num2str(port));
      | |ms=eval(get_param(gcb,'ms'));
      | set_param([gcb,'/tcp_ip_r'],'DataSize',['[',num2str(ms),']']);|Ts=eval(get_param(gcb,'Ts'));
      | set_param([gcb,'/tcp_ip_r'],'SampleTime',num2str(Ts));
  Plant_2_v : Subsystem  Orientation=left  AncestorBlock=passive_control/udp_nb_local_host  mask{port=9201}
      mask prompts: port "Port: [port]"
      mask CallbackString:
      | port=eval(get_param(gcb,'port'));
      | set_param([gcb,'/udp_s'],'Port',num2str(port));
  Plant_3_u : Subsystem  Orientation=left  AncestorBlock=passive_control/tcp_ip_nb_local_host  mask{port=9102, ms=3, Ts=0.05}
      mask prompts: port "Port: [port]"; ms "Vector length: [ms]"; Ts "Block sample time: [Ts]"
      mask CallbackString:
      | port=eval(get_param(gcb,'port'));
      | set_param([gcb,'/tcp_ip_r'],'Port',num2str(port));
      | |ms=eval(get_param(gcb,'ms'));
      | set_param([gcb,'/tcp_ip_r'],'DataSize',['[',num2str(ms),']']);|Ts=eval(get_param(gcb,'Ts'));
      | set_param([gcb,'/tcp_ip_r'],'SampleTime',num2str(Ts));
  Plant_3_v : Subsystem  Orientation=left  AncestorBlock=passive_control/udp_nb_local_host  mask{port=9202}
      mask prompts: port "Port: [port]"
      mask CallbackString:
      | port=eval(get_param(gcb,'port'));
      | set_param([gcb,'/udp_s'],'Port',num2str(port));
  avg_pj : passive_control/avg_pj  Orientation=left  SystemSampleTime=-1  np=2  nc=1  ms=3  Ts=.05
  rt_clock_f_mdl : passive_control/rt_clock_f_mdl  SystemSampleTime=-1  Ts=Ts  ID=ID
  t : Outport
  wires:
  rt_clock_f_mdl/1 -> t/1
  avg_pj/2 -> Plant_3_v/1(In1)
  avg_pj/3 -> Controller_1_u/1(In1)
  avg_pj/1 -> Plant_2_v/1(In1)
  Controller_1_v/2(data) -> avg_pj/6
  Controller_1_v/1(status) -> avg_pj/5
  Plant_3_u/2(data) -> avg_pj/4
  Plant_3_u/1(status) -> avg_pj/3
  Plant_2_u/2(data) -> avg_pj/2
  Plant_2_u/1(status) -> avg_pj/1

== system passive_control/passify ==
  theta : Inport
  Demux3 : Demux
  Mux7 : Mux
  ipesh_vel_est_1 : Subsystem  AncestorBlock=passive_control/ipesh_abcd  mask{num=[1,0], den=[tau,1], Ts=Ts, xp0=0}
      mask prompts: num "Enter num of H(s) [num]"; den "Enter den of H(s) [den]"; Ts "Enter sample time (s) [Ts]"; xp0 "Initial Joint Angle [xp0]"
      mask init:
      | Hs=tf(num,den);
      | Hz=ipesh_transform(Hs,Ts);
      | [A,B,C,D]=tf2ss(Hz.num{1},Hz.den{1})
      | [m,n]=size(A);
      | x0=-(D/(C))*xp0;
  ipesh_vel_est_2 : Subsystem  AncestorBlock=passive_control/ipesh_abcd  mask{num=[1,0], den=[tau,1], Ts=Ts, xp0=0}
      mask prompts: num "Enter num of H(s) [num]"; den "Enter den of H(s) [den]"; Ts "Enter sample time (s) [Ts]"; xp0 "Initial Joint Angle [xp0]"
      mask init:
      | Hs=tf(num,den);
      | Hz=ipesh_transform(Hs,Ts);
      | [A,B,C,D]=tf2ss(Hz.num{1},Hz.den{1})
      | [m,n]=size(A);
      | x0=-(D/(C))*xp0;
  ipesh_vel_est_3 : Subsystem  AncestorBlock=passive_control/ipesh_abcd  mask{num=[1,0], den=[tau,1], Ts=Ts, xp0=0}
      mask prompts: num "Enter num of H(s) [num]"; den "Enter den of H(s) [den]"; Ts "Enter sample time (s) [Ts]"; xp0 "Initial Joint Angle [xp0]"
      mask init:
      | Hs=tf(num,den);
      | Hz=ipesh_transform(Hs,Ts);
      | [A,B,C,D]=tf2ss(Hz.num{1},Hz.den{1})
      | [m,n]=size(A);
      | x0=-(D/(C))*xp0;
  ipesh_vel_est_4 : Subsystem  AncestorBlock=passive_control/ipesh_abcd  mask{num=[1,0], den=[tau,1], Ts=Ts, xp0=0}
      mask prompts: num "Enter num of H(s) [num]"; den "Enter den of H(s) [den]"; Ts "Enter sample time (s) [Ts]"; xp0 "Initial Joint Angle [xp0]"
      mask init:
      | Hs=tf(num,den);
      | Hz=ipesh_transform(Hs,Ts);
      | [A,B,C,D]=tf2ss(Hz.num{1},Hz.den{1})
      | [m,n]=size(A);
      | x0=-(D/(C))*xp0;
  omega : Outport
  wires:
  ipesh_vel_est_4/1(y) -> Mux7/4
  ipesh_vel_est_3/1(y) -> Mux7/3
  ipesh_vel_est_2/1(y) -> Mux7/2
  ipesh_vel_est_1/1(y) -> Mux7/1
  Mux7/1 -> omega/1
  theta/1 -> Demux3/1
  Demux3/4 -> ipesh_vel_est_4/1(u)
  Demux3/3 -> ipesh_vel_est_3/1(u)
  Demux3/2 -> ipesh_vel_est_2/1(u)
  Demux3/1 -> ipesh_vel_est_1/1(u)

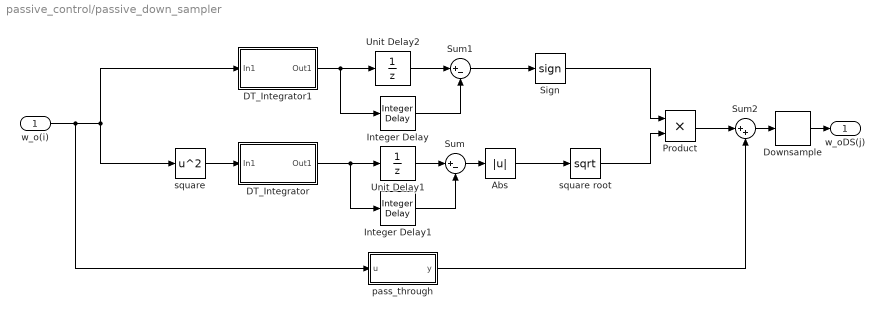
== system passive_control/passive_down_sampler ==
  w_o(i) : Inport  OutDataType=sfix(16)  OutScaling=2^0
  Abs : Abs  OutDataType=sfix(16)  OutScaling=2^0
  DT_Integrator : Subsystem
  DT_Integrator1 : Subsystem
  Downsample : dspsigops/Downsample  N=int16(M)  phase=0  ic=0  smode=Allow multirate  fmode=Maintain input frame size
  Integer Delay : simulink/Discrete/Integer Delay  vinit=0.0  samptime=-1  NumDelays=M
  Integer Delay1 : simulink/Discrete/Integer Delay  vinit=0.0  samptime=-1  NumDelays=M
  Product : Product  OutDataType=sfix(16)  OutScaling=2^0  RndMeth=Zero
  Sign : Signum
  Sum : Sum  Inputs=|+-  OutDataType=sfix(16)  OutScaling=2^0
  Sum1 : Sum  Inputs=|+-  OutDataType=sfix(16)  OutScaling=2^0
  Sum2 : Sum  Inputs=|++  OutDataType=sfix(16)  OutScaling=2^0
  Unit Delay1 : UnitDelay  SampleTime=-1
  Unit Delay2 : UnitDelay  SampleTime=-1
  pass_through : Stateflow chart
  square : Math  Operator=square  OutDataType=sfix(16)  OutScaling=2^0  SaturateOnIntegerOverflow=on
  square root : Math  Operator=sqrt  OutDataType=sfix(16)  OutScaling=2^0  SaturateOnIntegerOverflow=on
  w_oDS(j) : Outport  OutDataType=sfix(16)  OutScaling=2^0
  wires:
  pass_through/1(y) -> Sum2/2
  Sum2/1 -> Downsample/1
  Abs/1 -> square root/1
  w_o(i)/1 -> pass_through/1(u), square/1, DT_Integrator1/1(In1)
  Sum1/1 -> Sign/1
  Integer Delay/1 -> Sum1/2
  DT_Integrator1/1(Out1) -> Integer Delay/1, Unit Delay2/1
  Integer Delay1/1 -> Sum/2
  DT_Integrator/1(Out1) -> Integer Delay1/1, Unit Delay1/1
  Sign/1 -> Product/1
  square/1 -> DT_Integrator/1(In1)
  Sum/1 -> Abs/1
  square root/1 -> Product/2
  Product/1 -> Sum2/1
  Unit Delay2/1 -> Sum1/1
  Unit Delay1/1 -> Sum/1
  Downsample/1 -> w_oDS(j)/1

== system passive_control/passive_up_sampler ==
  w_iDS(j) : Inport  OutDataType=sfix(16)  OutScaling=2^0
  Gain : Gain  Gain=1.0/sqrt(M)  ParameterDataType=sfix(16)  ParameterScaling=2^0  OutDataType=sfix(16)  OutScaling=2^0
  M_sample_hold : Stateflow chart
  Unit Delay1 : UnitDelay  SampleTime=-1
  Upsample : dspsigops/Upsample  N=int16(M)  phase=0  ic=0  mode=Maintain input frame size
  w_i(i) : Outport  OutDataType=sfix(16)  OutScaling=2^0
  wires:
  M_sample_hold/1(y) -> w_i(i)/1
  Upsample/1 -> M_sample_hold/1(u)
  Unit Delay1/1 -> Gain/1
  w_iDS(j)/1 -> Unit Delay1/1
  Gain/1 -> Upsample/1

== system passive_control/rt_clock_f_mdl ==
  rt_clock_f_m : S-Function  FunctionName=rt_clock_f  Parameters=ID,Ts  EnableBusSupport=off
  scope : Scope
      settings: YMin=-0.045  YMax=0.015  SaveName=ScopeData7  MaxDataPoints=10
  t : Outport  OutDataType=sfix(16)  OutScaling=2^0
  wires:
  rt_clock_f_m/1 -> scope/1, t/1

== system passive_control/tcp_ip_nb_local_host ==
  tcp_ip_r : instrumentlib/TCP//IP Receive  Orientation=left  DialogController=instrumentcreatedialog  DialogControllerArgs=DataTag6  Host=127.0.0.1  Port=10000  DataSize=[3]  EnableBlockingMode=off  Timeout=10  SampleTime=0.05  DataType=double  ByteOrder=LittleEndian
  status : Outport  Orientation=left
  data : Outport  Orientation=left  Port=2
  wires:
  tcp_ip_r/1 -> data/1
  tcp_ip_r/2 -> status/1

== system passive_control/time_stamp ==
  u : Inport
  time_stamp : Stateflow chart
  y : Outport
  wires:
  u/1 -> time_stamp/1(u)
  time_stamp/1(y) -> y/1

== system passive_control/trajectory_gen ==
  theta : Inport
  Demux3 : Demux
  Mux7 : Mux
  ipesh_traj : Subsystem  AncestorBlock=passive_control/ipesh_abcd  mask{num=[wn^2], den=[1,2*zeta*wn,wn^2], Ts=Ts, xp0=[0,0]}
      mask prompts: num "Enter num of H(s) [num]"; den "Enter den of H(s) [den]"; Ts "Enter sample time (s) [Ts]"; xp0 "Initial Joint Angle [xp0]"
      mask init:
      | Hs=tf(num,den);
      | Hz=ipesh_transform(Hs,Ts);
      | [A,B,C,D]=tf2ss(Hz.num{1},Hz.den{1})
      | [m,n]=size(A);
      | x0=zeros(n,1);
  ipesh_traj1 : Subsystem  AncestorBlock=passive_control/ipesh_abcd  mask{num=[wn^2], den=[1,2*zeta*wn,wn^2], Ts=Ts, xp0=[0,0]}
      mask prompts: num "Enter num of H(s) [num]"; den "Enter den of H(s) [den]"; Ts "Enter sample time (s) [Ts]"; xp0 "Initial Joint Angle [xp0]"
      mask init:
      | Hs=tf(num,den);
      | Hz=ipesh_transform(Hs,Ts);
      | [A,B,C,D]=tf2ss(Hz.num{1},Hz.den{1})
      | [m,n]=size(A);
      | x0=zeros(n,1);
  ipesh_traj2 : Subsystem  AncestorBlock=passive_control/ipesh_abcd  mask{num=[wn^2], den=[1,2*zeta*wn,wn^2], Ts=Ts, xp0=[0,0]}
      mask prompts: num "Enter num of H(s) [num]"; den "Enter den of H(s) [den]"; Ts "Enter sample time (s) [Ts]"; xp0 "Initial Joint Angle [xp0]"
      mask init:
      | Hs=tf(num,den);
      | Hz=ipesh_transform(Hs,Ts);
      | [A,B,C,D]=tf2ss(Hz.num{1},Hz.den{1})
      | [m,n]=size(A);
      | x0=zeros(n,1);
  ipesh_traj3 : Subsystem  AncestorBlock=passive_control/ipesh_abcd  mask{num=[wn^2], den=[1,2*zeta*wn,wn^2], Ts=Ts, xp0=[0,0]}
      mask prompts: num "Enter num of H(s) [num]"; den "Enter den of H(s) [den]"; Ts "Enter sample time (s) [Ts]"; xp0 "Initial Joint Angle [xp0]"
      mask init:
      | Hs=tf(num,den);
      | Hz=ipesh_transform(Hs,Ts);
      | [A,B,C,D]=tf2ss(Hz.num{1},Hz.den{1})
      | [m,n]=size(A);
      | x0=zeros(n,1);
  omega : Outport
  wires:
  Demux3/1 -> ipesh_traj/1(u)
  Demux3/2 -> ipesh_traj1/1(u)
  Demux3/3 -> ipesh_traj2/1(u)
  Demux3/4 -> ipesh_traj3/1(u)
  theta/1 -> Demux3/1
  Mux7/1 -> omega/1
  ipesh_traj/1(y) -> Mux7/1
  ipesh_traj1/1(y) -> Mux7/2
  ipesh_traj2/1(y) -> Mux7/3
  ipesh_traj3/1(y) -> Mux7/4

== system passive_control/udp_nb_local_host ==
  In1 : Inport  Orientation=left
  udp_s : instrumentlib/UDP Send  Orientation=left  DialogController=instrumentcreatedialog  DialogControllerArgs=DataTag7  Host=127.0.0.1  Port=9001  LocalPort=-1  EnableBlockingMode=off  ByteOrder=LittleEndian
  wires:
  In1/1 -> udp_s/1

== system passive_control/Crustcrawler Robot/vel_est ==
  theta : Inport
  Demux3 : Demux
  Mux7 : Mux
  ipesh_vel_est_1 : Subsystem  AncestorBlock=passive_control/ipesh_abcd  mask{num=[1 0], den=[.1/pi 1], Ts=.04, xp0=0}
      mask prompts: num "Enter num of H(s) [num]"; den "Enter den of H(s) [den]"; Ts "Enter sample time (s) [Ts]"; xp0 "Initial Joint Angle [xp0]"
      mask init:
      | Hs=tf(num,den);
      | Hz=ipesh_transform(Hs,Ts);
      | [A,B,C,D]=tf2ss(Hz.num{1},Hz.den{1})
      | [m,n]=size(A);
      | x0=-(D/(C))*xp0;
  ipesh_vel_est_2 : Subsystem  AncestorBlock=passive_control/ipesh_abcd  mask{num=[1 0], den=[.1/pi 1], Ts=.04, xp0=-pi/2}
      mask prompts: num "Enter num of H(s) [num]"; den "Enter den of H(s) [den]"; Ts "Enter sample time (s) [Ts]"; xp0 "Initial Joint Angle [xp0]"
      mask init:
      | Hs=tf(num,den);
      | Hz=ipesh_transform(Hs,Ts);
      | [A,B,C,D]=tf2ss(Hz.num{1},Hz.den{1})
      | [m,n]=size(A);
      | x0=-(D/(C))*xp0;
  ipesh_vel_est_3 : Subsystem  AncestorBlock=passive_control/ipesh_abcd  mask{num=[1 0], den=[.1/pi 1], Ts=.04, xp0=pi/2}
      mask prompts: num "Enter num of H(s) [num]"; den "Enter den of H(s) [den]"; Ts "Enter sample time (s) [Ts]"; xp0 "Initial Joint Angle [xp0]"
      mask init:
      | Hs=tf(num,den);
      | Hz=ipesh_transform(Hs,Ts);
      | [A,B,C,D]=tf2ss(Hz.num{1},Hz.den{1})
      | [m,n]=size(A);
      | x0=-(D/(C))*xp0;
  ipesh_vel_est_4 : Subsystem  AncestorBlock=passive_control/ipesh_abcd  mask{num=[1 0], den=[.1/pi 1], Ts=.04, xp0=0}
      mask prompts: num "Enter num of H(s) [num]"; den "Enter den of H(s) [den]"; Ts "Enter sample time (s) [Ts]"; xp0 "Initial Joint Angle [xp0]"
      mask init:
      | Hs=tf(num,den);
      | Hz=ipesh_transform(Hs,Ts);
      | [A,B,C,D]=tf2ss(Hz.num{1},Hz.den{1})
      | [m,n]=size(A);
      | x0=-(D/(C))*xp0;
  omega : Outport
  wires:
  ipesh_vel_est_4/1(y) -> Mux7/4
  ipesh_vel_est_3/1(y) -> Mux7/3
  ipesh_vel_est_2/1(y) -> Mux7/2
  ipesh_vel_est_1/1(y) -> Mux7/1
  Mux7/1 -> omega/1
  theta/1 -> Demux3/1
  Demux3/4 -> ipesh_vel_est_4/1(u)
  Demux3/3 -> ipesh_vel_est_3/1(u)
  Demux3/2 -> ipesh_vel_est_2/1(u)
  Demux3/1 -> ipesh_vel_est_1/1(u)

== system passive_control/Kp_Kv_CrustCrawler/trajectory_gen ==
  theta : Inport
  Demux3 : Demux
  Mux7 : Mux
  ipesh_traj : Subsystem  AncestorBlock=passive_control/ipesh_abcd  mask{num=[wn^2], den=[1,2*zeta*wn,wn^2], Ts=Ts, xp0=[0,0]}
      mask prompts: num "Enter num of H(s) [num]"; den "Enter den of H(s) [den]"; Ts "Enter sample time (s) [Ts]"; xp0 "Initial Joint Angle [xp0]"
      mask init:
      | Hs=tf(num,den);
      | Hz=ipesh_transform(Hs,Ts);
      | [A,B,C,D]=tf2ss(Hz.num{1},Hz.den{1})
      | [m,n]=size(A);
      | x0=zeros(n,1);
  ipesh_traj1 : Subsystem  AncestorBlock=passive_control/ipesh_abcd  mask{num=[wn^2], den=[1,2*zeta*wn,wn^2], Ts=Ts, xp0=[0,0]}
      mask prompts: num "Enter num of H(s) [num]"; den "Enter den of H(s) [den]"; Ts "Enter sample time (s) [Ts]"; xp0 "Initial Joint Angle [xp0]"
      mask init:
      | Hs=tf(num,den);
      | Hz=ipesh_transform(Hs,Ts);
      | [A,B,C,D]=tf2ss(Hz.num{1},Hz.den{1})
      | [m,n]=size(A);
      | x0=zeros(n,1);
  ipesh_traj2 : Subsystem  AncestorBlock=passive_control/ipesh_abcd  mask{num=[wn^2], den=[1,2*zeta*wn,wn^2], Ts=Ts, xp0=[0,0]}
      mask prompts: num "Enter num of H(s) [num]"; den "Enter den of H(s) [den]"; Ts "Enter sample time (s) [Ts]"; xp0 "Initial Joint Angle [xp0]"
      mask init:
      | Hs=tf(num,den);
      | Hz=ipesh_transform(Hs,Ts);
      | [A,B,C,D]=tf2ss(Hz.num{1},Hz.den{1})
      | [m,n]=size(A);
      | x0=zeros(n,1);
  ipesh_traj3 : Subsystem  AncestorBlock=passive_control/ipesh_abcd  mask{num=[wn^2], den=[1,2*zeta*wn,wn^2], Ts=Ts, xp0=[0,0]}
      mask prompts: num "Enter num of H(s) [num]"; den "Enter den of H(s) [den]"; Ts "Enter sample time (s) [Ts]"; xp0 "Initial Joint Angle [xp0]"
      mask init:
      | Hs=tf(num,den);
      | Hz=ipesh_transform(Hs,Ts);
      | [A,B,C,D]=tf2ss(Hz.num{1},Hz.den{1})
      | [m,n]=size(A);
      | x0=zeros(n,1);
  omega : Outport
  wires:
  Demux3/1 -> ipesh_traj/1(u)
  Demux3/2 -> ipesh_traj1/1(u)
  Demux3/3 -> ipesh_traj2/1(u)
  Demux3/4 -> ipesh_traj3/1(u)
  theta/1 -> Demux3/1
  Mux7/1 -> omega/1
  ipesh_traj/1(y) -> Mux7/1
  ipesh_traj1/1(y) -> Mux7/2
  ipesh_traj2/1(y) -> Mux7/3
  ipesh_traj3/1(y) -> Mux7/4

== system passive_control/Kp_Kv_CrustCrawler/vel_est ==
  theta : Inport
  Demux3 : Demux
  Mux7 : Mux
  ipesh_vel_est_1 : Subsystem  AncestorBlock=passive_control/ipesh_abcd  mask{num=[1 0], den=[Ts/pi 1], Ts=Ts, xp0=q0(1)}
      mask prompts: num "Enter num of H(s) [num]"; den "Enter den of H(s) [den]"; Ts "Enter sample time (s) [Ts]"; xp0 "Initial Joint Angle [xp0]"
      mask init:
      | Hs=tf(num,den);
      | Hz=ipesh_transform(Hs,Ts);
      | [A,B,C,D]=tf2ss(Hz.num{1},Hz.den{1})
      | [m,n]=size(A);
      | x0=-(D/(C))*xp0;
  ipesh_vel_est_2 : Subsystem  AncestorBlock=passive_control/ipesh_abcd  mask{num=[1 0], den=[Ts/pi 1], Ts=Ts, xp0=q0(2)}
      mask prompts: num "Enter num of H(s) [num]"; den "Enter den of H(s) [den]"; Ts "Enter sample time (s) [Ts]"; xp0 "Initial Joint Angle [xp0]"
      mask init:
      | Hs=tf(num,den);
      | Hz=ipesh_transform(Hs,Ts);
      | [A,B,C,D]=tf2ss(Hz.num{1},Hz.den{1})
      | [m,n]=size(A);
      | x0=-(D/(C))*xp0;
  ipesh_vel_est_3 : Subsystem  AncestorBlock=passive_control/ipesh_abcd  mask{num=[1 0], den=[Ts/pi 1], Ts=Ts, xp0=q0(3)}
      mask prompts: num "Enter num of H(s) [num]"; den "Enter den of H(s) [den]"; Ts "Enter sample time (s) [Ts]"; xp0 "Initial Joint Angle [xp0]"
      mask init:
      | Hs=tf(num,den);
      | Hz=ipesh_transform(Hs,Ts);
      | [A,B,C,D]=tf2ss(Hz.num{1},Hz.den{1})
      | [m,n]=size(A);
      | x0=-(D/(C))*xp0;
  ipesh_vel_est_4 : Subsystem  AncestorBlock=passive_control/ipesh_abcd  mask{num=[1 0], den=[Ts/pi 1], Ts=Ts, xp0=q0(4)}
      mask prompts: num "Enter num of H(s) [num]"; den "Enter den of H(s) [den]"; Ts "Enter sample time (s) [Ts]"; xp0 "Initial Joint Angle [xp0]"
      mask init:
      | Hs=tf(num,den);
      | Hz=ipesh_transform(Hs,Ts);
      | [A,B,C,D]=tf2ss(Hz.num{1},Hz.den{1})
      | [m,n]=size(A);
      | x0=-(D/(C))*xp0;
  omega : Outport
  wires:
  Demux3/1 -> ipesh_vel_est_1/1(u)
  Demux3/2 -> ipesh_vel_est_2/1(u)
  Demux3/3 -> ipesh_vel_est_3/1(u)
  Demux3/4 -> ipesh_vel_est_4/1(u)
  theta/1 -> Demux3/1
  Mux7/1 -> omega/1
  ipesh_vel_est_1/1(y) -> Mux7/1
  ipesh_vel_est_2/1(y) -> Mux7/2
  ipesh_vel_est_3/1(y) -> Mux7/3
  ipesh_vel_est_4/1(y) -> Mux7/4

== system passive_control/cc_wave_filter/ipesh_abcd ==
  u : Inport
  Embedded MATLAB Function : Stateflow chart
  Unit Delay : UnitDelay  Orientation=left  X0=x0  SampleTime=-1
  y : Outport
  wires:
  Embedded MATLAB Function/1(y) -> y/1
  u/1 -> Embedded MATLAB Function/1(u)
  Unit Delay/1 -> Embedded MATLAB Function/2(x_k)
  Embedded MATLAB Function/2(x_k_p_1) -> Unit Delay/1

== system passive_control/cc_wave_filter/ipesh_abcd1 ==
  u : Inport
  Embedded MATLAB Function : Stateflow chart
  Unit Delay : UnitDelay  Orientation=left  X0=x0  SampleTime=-1
  y : Outport
  wires:
  Embedded MATLAB Function/2(x_k_p_1) -> Unit Delay/1
  Unit Delay/1 -> Embedded MATLAB Function/2(x_k)
  u/1 -> Embedded MATLAB Function/1(u)
  Embedded MATLAB Function/1(y) -> y/1

== system passive_control/cc_wave_filter/ipesh_abcd2 ==
  u : Inport
  Embedded MATLAB Function : Stateflow chart
  Unit Delay : UnitDelay  Orientation=left  X0=x0  SampleTime=-1
  y : Outport
  wires:
  Embedded MATLAB Function/1(y) -> y/1
  u/1 -> Embedded MATLAB Function/1(u)
  Unit Delay/1 -> Embedded MATLAB Function/2(x_k)
  Embedded MATLAB Function/2(x_k_p_1) -> Unit Delay/1

== system passive_control/cc_wave_filter/ipesh_abcd3 ==
  u : Inport
  Embedded MATLAB Function : Stateflow chart
  Unit Delay : UnitDelay  Orientation=left  X0=x0  SampleTime=-1
  y : Outport
  wires:
  Embedded MATLAB Function/2(x_k_p_1) -> Unit Delay/1
  Unit Delay/1 -> Embedded MATLAB Function/2(x_k)
  u/1 -> Embedded MATLAB Function/1(u)
  Embedded MATLAB Function/1(y) -> y/1

== system passive_control/lag_compensator/lag_compen ==
  u : Inport
  Embedded MATLAB Function : Stateflow chart
  Unit Delay : UnitDelay  X0=x0  SampleTime=-1
  y : Outport
  wires:
  Embedded MATLAB Function/2(x_k_p_1) -> Unit Delay/1
  Unit Delay/1 -> Embedded MATLAB Function/2(x_k)
  u/1 -> Embedded MATLAB Function/1(u)
  Embedded MATLAB Function/1(y) -> y/1

== system passive_control/lag_compensator/lag_compen1 ==
  u : Inport
  Embedded MATLAB Function : Stateflow chart
  Unit Delay : UnitDelay  X0=x0  SampleTime=-1
  y : Outport
  wires:
  Embedded MATLAB Function/1(y) -> y/1
  u/1 -> Embedded MATLAB Function/1(u)
  Unit Delay/1 -> Embedded MATLAB Function/2(x_k)
  Embedded MATLAB Function/2(x_k_p_1) -> Unit Delay/1

== system passive_control/lag_compensator/lag_compen2 ==
  u : Inport
  Embedded MATLAB Function : Stateflow chart
  Unit Delay : UnitDelay  X0=x0  SampleTime=-1
  y : Outport
  wires:
  Embedded MATLAB Function/2(x_k_p_1) -> Unit Delay/1
  Unit Delay/1 -> Embedded MATLAB Function/2(x_k)
  u/1 -> Embedded MATLAB Function/1(u)
  Embedded MATLAB Function/1(y) -> y/1

== system passive_control/lag_compensator/lag_compen3 ==
  u : Inport
  Embedded MATLAB Function : Stateflow chart
  Unit Delay : UnitDelay  X0=x0  SampleTime=-1
  y : Outport
  wires:
  Embedded MATLAB Function/1(y) -> y/1
  u/1 -> Embedded MATLAB Function/1(u)
  Unit Delay/1 -> Embedded MATLAB Function/2(x_k)
  Embedded MATLAB Function/2(x_k_p_1) -> Unit Delay/1

== system passive_control/net_avg_pj/Controller_1_u ==
  In1 : Inport  Orientation=left
  udp_s : instrumentlib/UDP Send  Orientation=left  DialogController=instrumentcreatedialog  DialogControllerArgs=DataTag0  Host=127.0.0.1  Port=9200  LocalPort=-1  EnableBlockingMode=off  ByteOrder=LittleEndian
  wires:
  In1/1 -> udp_s/1

== system passive_control/net_avg_pj/Controller_1_v ==
  tcp_ip_r : instrumentlib/TCP//IP Receive  Orientation=left  DialogController=instrumentcreatedialog  DialogControllerArgs=DataTag1  Host=127.0.0.1  Port=9100  DataSize=[3]  EnableBlockingMode=off  Timeout=10  SampleTime=0.05  DataType=double  ByteOrder=LittleEndian
  status : Outport  Orientation=left
  data : Outport  Orientation=left  Port=2
  wires:
  tcp_ip_r/1 -> data/1
  tcp_ip_r/2 -> status/1

== system passive_control/net_avg_pj/Plant_2_u ==
  tcp_ip_r : instrumentlib/TCP//IP Receive  Orientation=left  DialogController=instrumentcreatedialog  DialogControllerArgs=DataTag2  Host=127.0.0.1  Port=9101  DataSize=[3]  EnableBlockingMode=off  Timeout=10  SampleTime=0.05  DataType=double  ByteOrder=LittleEndian
  status : Outport  Orientation=left
  data : Outport  Orientation=left  Port=2
  wires:
  tcp_ip_r/1 -> data/1
  tcp_ip_r/2 -> status/1

== system passive_control/net_avg_pj/Plant_2_v ==
  In1 : Inport  Orientation=left
  udp_s : instrumentlib/UDP Send  Orientation=left  DialogController=instrumentcreatedialog  DialogControllerArgs=DataTag3  Host=127.0.0.1  Port=9201  LocalPort=-1  EnableBlockingMode=off  ByteOrder=LittleEndian
  wires:
  In1/1 -> udp_s/1

== system passive_control/net_avg_pj/Plant_3_u ==
  tcp_ip_r : instrumentlib/TCP//IP Receive  Orientation=left  DialogController=instrumentcreatedialog  DialogControllerArgs=DataTag4  Host=127.0.0.1  Port=9102  DataSize=[3]  EnableBlockingMode=off  Timeout=10  SampleTime=0.05  DataType=double  ByteOrder=LittleEndian
  status : Outport  Orientation=left
  data : Outport  Orientation=left  Port=2
  wires:
  tcp_ip_r/2 -> status/1
  tcp_ip_r/1 -> data/1

== system passive_control/net_avg_pj/Plant_3_v ==
  In1 : Inport  Orientation=left
  udp_s : instrumentlib/UDP Send  Orientation=left  DialogController=instrumentcreatedialog  DialogControllerArgs=DataTag5  Host=127.0.0.1  Port=9202  LocalPort=-1  EnableBlockingMode=off  ByteOrder=LittleEndian
  wires:
  In1/1 -> udp_s/1

== system passive_control/passify/ipesh_vel_est_1 ==
  u : Inport
  Embedded MATLAB Function : Stateflow chart
  Unit Delay : UnitDelay  X0=x0  SampleTime=-1
  y : Outport
  wires:
  Embedded MATLAB Function/2(x_k_p_1) -> Unit Delay/1
  Unit Delay/1 -> Embedded MATLAB Function/2(x_k)
  u/1 -> Embedded MATLAB Function/1(u)
  Embedded MATLAB Function/1(y) -> y/1
